simulink model "simrotor3a"  (Simulink 3.00)
settings: Solver=ode23tb  SolverMode=SingleTasking  StartTime=0.0  StopTime=50  RelTol=1e-2  AbsTol=1e-2
libraries: simulink3 x1

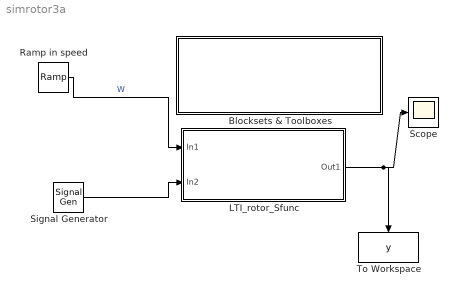
== system simrotor3a ==
  Blocksets & Toolboxes : Subsystem
      settings: OpenFcn=clf,drawrot simple1
      mask Display: fprintf(' example for simulating a \n Speed varying torsionaly stiff rotor\n')
  LTI_rotor_Sfunc : Subsystem  mask{Model=simple1s}
      mask prompts: Model "Model Template File"
      mask help: Sfunction accepts a template file + speed
      mask init:
      | Rot=rotfe(Model);
      mask Display: disp(Model)
  Ramp in speed : simulink3/Sources/Ramp  slope=30*2*pi/60/10  start=0  X0=0
  Scope : Scope
      settings: TickLabels=on  TimeRange=auto  YMin=-0.075  YMax=0.075  SaveToWorkspace=off  SaveName=ScopeData  DataFormat=Matrix
  Signal Generator : SignalGenerator  WaveForm=square  Amplitude=1  Frequency=.20  Units=Hertz
  To Workspace : ToWorkspace  VariableName=y  SampleTime=1/50  SaveFormat=Matrix
      settings: Orientation=down
  wires:
  Signal Generator/1 -> LTI_rotor_Sfunc/2(In2)
  LTI_rotor_Sfunc/1(Out1) -> Scope/1, To Workspace/1
  Ramp in speed/1 -> LTI_rotor_Sfunc/1(In1)  "W"

== system simrotor3a/Blocksets & Toolboxes ==

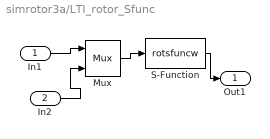
== system simrotor3a/LTI_rotor_Sfunc ==
  In1 : Inport  Port=1  PortWidth=-1  SampleTime=-1  DataType=auto
      settings: SignalType=auto
  In2 : Inport  Port=2  PortWidth=-1  SampleTime=-1  DataType=auto
      settings: SignalType=auto
  Mux : Mux  Inputs=2
      settings: DisplayOption=none
  S-Function : S-Function  FunctionName=rotsfuncw  Parameters=Rot  PortCounts=[]  SFunctionModules=''
  Out1 : Outport  Port=1
  wires:
  S-Function/1 -> Out1/1
  Mux/1 -> S-Function/1
  In1/1 -> Mux/1
  In2/1 -> Mux/2
